simulink model "Lab1_ex2_i"  (R2021b)
settings: Solver=VariableStepAuto  StartTime=0.0  StopTime=100  RelTol=1e-3
libraries: simulink x1
settings Model: Creator=pacur  LastModifiedBy=pacur

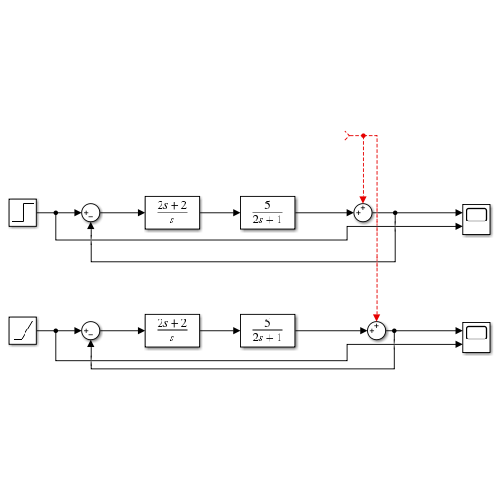
[thumbnail: Simulink's stored preview of the top-level diagram]
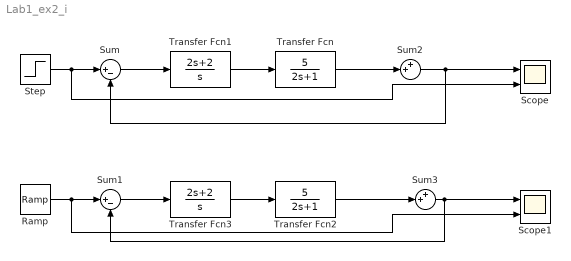
== system Lab1_ex2_i ==
  Ramp : simulink/Sources/Ramp  slope=1  start=0  InitialOutput=0
  Scope : Scope  NumInputPorts=2
  Scope1 : Scope  NumInputPorts=2
  Step : Step  SampleTime=0
  Sum : Sum  Inputs=|+-
  Sum1 : Sum  Inputs=|+-
  Sum2 : Sum  Inputs=++|
  Sum3 : Sum  Inputs=++|
  Transfer Fcn : TransferFcn  Numerator=[5]  Denominator=[2 1]
  Transfer Fcn1 : TransferFcn  Numerator=[2 2]  Denominator=[1 0]
  Transfer Fcn2 : TransferFcn  Numerator=[5]  Denominator=[2 1]
  Transfer Fcn3 : TransferFcn  Numerator=[2 2]  Denominator=[1 0]
  wires:
  Step/1 -> Scope/2, Sum/1
  Transfer Fcn1/1 -> Transfer Fcn/1
  Sum/1 -> Transfer Fcn1/1
  Transfer Fcn/1 -> Sum2/2
  Transfer Fcn3/1 -> Transfer Fcn2/1
  Sum1/1 -> Transfer Fcn3/1
  Ramp/1 -> Scope1/2, Sum1/1
  Sum2/1 -> Sum/2, Scope/1
  Transfer Fcn2/1 -> Sum3/2
  Sum3/1 -> Scope1/1, Sum1/2
  ? -> Sum3/1, Sum2/1
